simulink model "Provaa"  (R2020a)
settings: Solver=VariableStepAuto  StartTime=0.0  StopTime=10.0  RelTol=1e-3
libraries: simulink x1
settings Model: Creator=cvalo  LastModifiedBy=cvalo

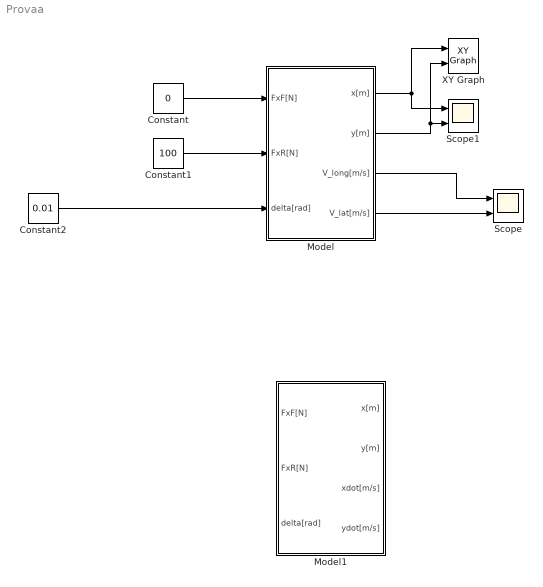
== system Provaa ==
  Constant : Constant  Value=0
  Constant1 : Constant  Value=100
  Constant2 : Constant  Value=0.01
  Model : Subsystem
  Model1 : Subsystem
  Scope : Scope  NumInputPorts=2
  Scope1 : Scope  NumInputPorts=2
  XY Graph : simulink/Sinks/XY Graph  xmin=-1  xmax=500  ymin=-10  ymax=250  st=-1
  wires:
  Model/3(V_long[m/s]) -> Scope/1
  Model/4(V_lat[m/s]) -> Scope/2
  Model/1(x[m]) -> Scope1/1, XY Graph/1
  Model/2(y[m]) -> XY Graph/2, Scope1/2
  Constant/1 -> Model/1(FxF[N])
  Constant1/1 -> Model/2(FxR[N])
  Constant2/1 -> Model/3(delta[rad])

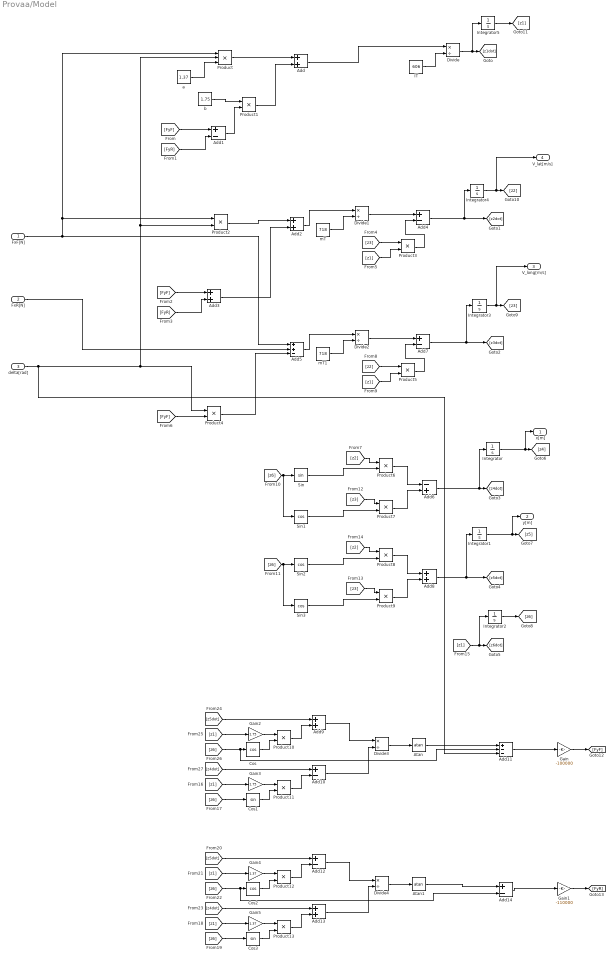
== system Provaa/Model ==
  FxF[N] : Inport  Unit=N
  FxR[N] : Inport  Port=2  Unit=N
  delta[rad] : Inport  Port=3  Unit=rad
  Add{,2..3,8..9,13} (6 alike) : Sum
  Add{1,4,7,10,12,14} (6 alike) : Sum  Inputs=+-
  Add11 : Sum  Inputs=+--
  Add5 : Sum  Inputs=++-
  Add6 : Sum  Inputs=-+
  Atan : Trigonometry  Operator=atan
  Atan1 : Trigonometry  Operator=atan
  Cos : Trigonometry  Operator=cos
  Cos1 : Trigonometry
  Cos2 : Trigonometry  Operator=cos
  Cos3 : Trigonometry
  Divide{,1..4} (5 alike) : Product  Inputs=*/
  Gain : Gain  Gain=-100000
  Gain1 : Gain  Gain=-110000
  Gain2 : Gain  Gain=1.75
  Gain3 : Gain  Gain=1.75
  Gain4 : Gain  Gain=1.37
  Gain5 : Gain  Gain=1.37
  IT : Constant  Value=606
  Integrator{,1..2,4..5} (5 alike) : Integrator
  Integrator3 : Integrator  InitialCondition=10
  Product : Product  Inputs=3
  Product{1..13} (13 alike) : Product
  Sin : Trigonometry
  Sin1 : Trigonometry  Operator=cos
  Sin2 : Trigonometry  Operator=cos
  Sin3 : Trigonometry  Operator=cos
  a : Constant  Value=1.37
  b : Constant  Value=1.75
  mT : Constant  Value=718
  mT1 : Constant  Value=718
  x[m] : Outport  Unit=m
  y[m] : Outport  Port=2  Unit=m
  V_long[m/s] : Outport  Port=3  Unit=m/s
  V_lat[m/s] : Outport  Port=4  Unit=m/s
  wires:
  Divide/1 -> Integrator5/1, [z1dot]
  IT/1 -> Divide/2
  a/1 -> Product/3
  Product/1 -> Add/1
  Product1/1 -> Add/2
  b/1 -> Product1/1
  Add1/1 -> Product1/2
  [FyF] -> Add1/1
  [FyR] -> Add1/2
  Add/1 -> Divide/1
  Add3/1 -> Add2/2
  [FyF] -> Add3/1
  Divide1/1 -> Add4/1
  Add2/1 -> Divide1/1
  [FyR] -> Add3/2
  mT/1 -> Divide1/2
  Product2/1 -> Add2/1
  Add4/1 -> Integrator4/1, [z2dot]
  Product3/1 -> Add4/2
  [z3] -> Product3/1
  [z1] -> Product3/2
  [z1] -> Product5/2
  FxF[N]/1 -> Add5/1, Product/1, Product2/1
  [FyF] -> Product4/2
  Product5/1 -> Add7/2
  Add5/1 -> Divide2/1
  Add7/1 -> Integrator3/1, [z3dot]
  Product4/1 -> Add5/3
  mT1/1 -> Divide2/2
  Divide2/1 -> Add7/1
  [z2] -> Product5/1
  FxR[N]/1 -> Add5/2
  Add6/1 -> Integrator/1, [z4dot]
  Product6/1 -> Add6/1
  Product7/1 -> Add6/2
  [z2] -> Product6/1
  Sin/1 -> Product6/2
  [z3] -> Product7/1
  Sin1/1 -> Product7/2
  [z6] -> Sin1/1, Sin/1
  Sin2/1 -> Product8/2
  Sin3/1 -> Product9/2
  Product8/1 -> Add8/1
  [z3] -> Product9/1
  Product9/1 -> Add8/2
  [z2] -> Product8/1
  [z6] -> Sin3/1, Sin2/1
  [z1] -> Integrator2/1, [z6dot]
  Integrator/1 -> x[m]/1, [z4]
  Integrator1/1 -> y[m]/1, [z5]
  Add8/1 -> [z5dot], Integrator1/1
  Integrator2/1 -> [z6]
  Integrator3/1 -> V_long[m/s]/1, [z3]
  Integrator4/1 -> V_lat[m/s]/1, [z2]
  Integrator5/1 -> [z1]
  Gain1/1 -> [FyR]
  Gain/1 -> [FyF]
  Atan/1 -> Add11/1
  Add9/1 -> Divide3/1
  Cos/1 -> Product10/2
  delta[rad]/1 -> Add11/3, Product4/1, Product/2, Product2/2
  [z4dot] -> Add10/1
  Add14/1 -> Gain1/1
  Cos3/1 -> Product13/2
  Divide3/1 -> Atan/1
  Product13/1 -> Add13/2
  Gain3/1 -> Product11/1
  Add10/1 -> Divide3/2
  [z5dot] -> Add9/1
  [z6] -> Cos1/1
  [z6] -> Add11/2, Cos/1
  [z6] -> Add14/2, Cos2/1
  Cos2/1 -> Product12/2
  [z1] -> Gain4/1
  Gain2/1 -> Product10/1
  Gain5/1 -> Product13/1
  Add11/1 -> Gain/1
  Divide4/1 -> Atan1/1
  Add12/1 -> Divide4/1
  [z1] -> Gain3/1
  Add13/1 -> Divide4/2
  Product10/1 -> Add9/2
  Cos1/1 -> Product11/2
  [z5dot] -> Add12/1
  Atan1/1 -> Add14/1
  [z1] -> Gain2/1
  [z6] -> Cos3/1
  Product11/1 -> Add10/2
  Product12/1 -> Add12/2
  [z1] -> Gain5/1
  Gain4/1 -> Product12/1
  [z4dot] -> Add13/1

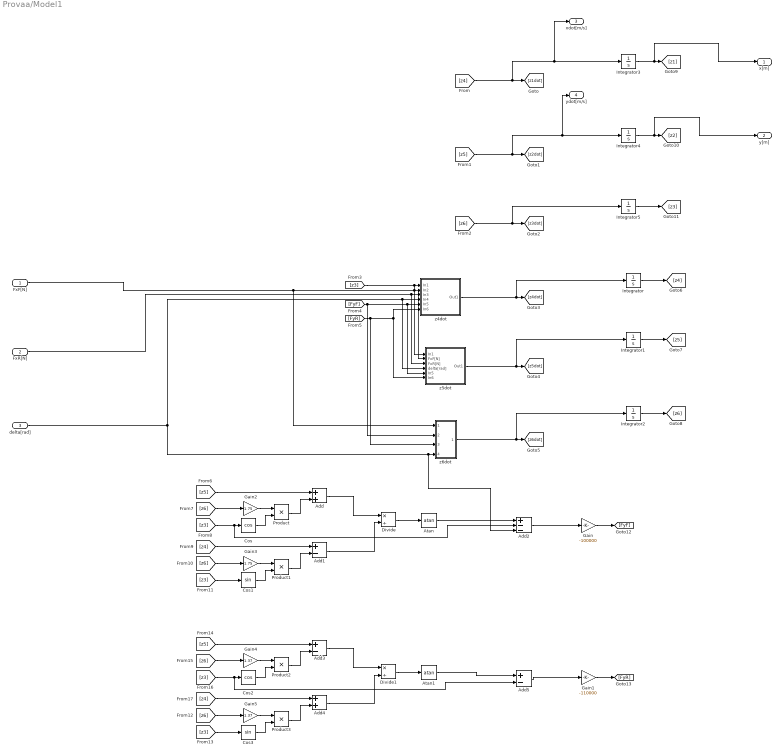
== system Provaa/Model1 ==
  FxF[N] : Inport  Unit=N
  FxR[N] : Inport  Port=2  Unit=N
  delta[rad] : Inport  Port=3  Unit=rad
  Add : Sum
  Add1 : Sum  Inputs=+-
  Add2 : Sum  Inputs=+--
  Add3 : Sum  Inputs=+-
  Add4 : Sum
  Add5 : Sum  Inputs=+-
  Atan : Trigonometry  Operator=atan
  Atan1 : Trigonometry  Operator=atan
  Cos : Trigonometry  Operator=cos
  Cos1 : Trigonometry
  Cos2 : Trigonometry  Operator=cos
  Cos3 : Trigonometry
  Divide : Product  Inputs=*/
  Divide1 : Product  Inputs=*/
  Gain : Gain  Gain=-100000
  Gain1 : Gain  Gain=-110000
  Gain2 : Gain  Gain=1.75
  Gain3 : Gain  Gain=1.75
  Gain4 : Gain  Gain=1.37
  Gain5 : Gain  Gain=1.37
  Integrator : Integrator  InitialCondition=10
  Integrator{1..5} (5 alike) : Integrator
  Product{,1..3} (4 alike) : Product
  z4dot : Subsystem
  z5dot : Subsystem
  z6dot : Subsystem
  x[m] : Outport  Unit=m
  y[m] : Outport  Port=2  Unit=m
  xdot[m/s] : Outport  Port=3  Unit=m/s
  ydot[m/s] : Outport  Port=4  Unit=m/s
  wires:
  [z3] -> z5dot/1(In1), z4dot/1(In1)
  FxF[N]/1 -> z6dot/1(In1), z5dot/2(FxF[N]), z4dot/2(In2)
  FxR[N]/1 -> z5dot/3(FxR[N]), z4dot/3(In3)
  delta[rad]/1 -> Add2/3, z6dot/4(In4), z4dot/4(In4), z5dot/4(delta[rad])
  [FyF] -> z6dot/2(In2), z4dot/5(In5), z5dot/5(In5)
  [FyR] -> z6dot/3(In3), z5dot/6(In6), z4dot/6(In6)
  z4dot/1(Out1) -> Integrator/1, [z4dot]
  Integrator/1 -> [z4]
  Integrator1/1 -> [z5]
  z5dot/1(Out1) -> Integrator1/1, [z5dot]
  Integrator2/1 -> [z6]
  z6dot/1(Out1) -> Integrator2/1, [z6dot]
  Integrator3/1 -> x[m]/1, [z1]
  [z4] -> xdot[m/s]/1, Integrator3/1, [z1dot]
  Integrator4/1 -> y[m]/1, [z2]
  [z5] -> ydot[m/s]/1, Integrator4/1, [z2dot]
  Integrator5/1 -> [z3]
  [z6] -> Integrator5/1, [z3dot]
  Gain/1 -> [FyF]
  Gain1/1 -> [FyR]
  Atan/1 -> Add2/1
  Divide/1 -> Atan/1
  [z5] -> Add/1
  Add/1 -> Divide/1
  [z6] -> Gain2/1
  Gain2/1 -> Product/1
  Cos/1 -> Product/2
  [z3] -> Add2/2, Cos/1
  Product/1 -> Add/2
  [z3] -> Cos1/1
  [z4] -> Add1/1
  Add1/1 -> Divide/2
  Product1/1 -> Add1/2
  Gain3/1 -> Product1/1
  [z6] -> Gain3/1
  Cos1/1 -> Product1/2
  Add2/1 -> Gain/1
  [z3] -> Add5/2, Cos2/1
  [z6] -> Gain5/1
  Add5/1 -> Gain1/1
  Product3/1 -> Add4/2
  Gain5/1 -> Product3/1
  Cos3/1 -> Product3/2
  [z4] -> Add4/1
  [z3] -> Cos3/1
  Atan1/1 -> Add5/1
  Add4/1 -> Divide1/2
  [z5] -> Add3/1
  Add3/1 -> Divide1/1
  Product2/1 -> Add3/2
  Gain4/1 -> Product2/1
  Divide1/1 -> Atan1/1
  [z6] -> Gain4/1
  Cos2/1 -> Product2/2

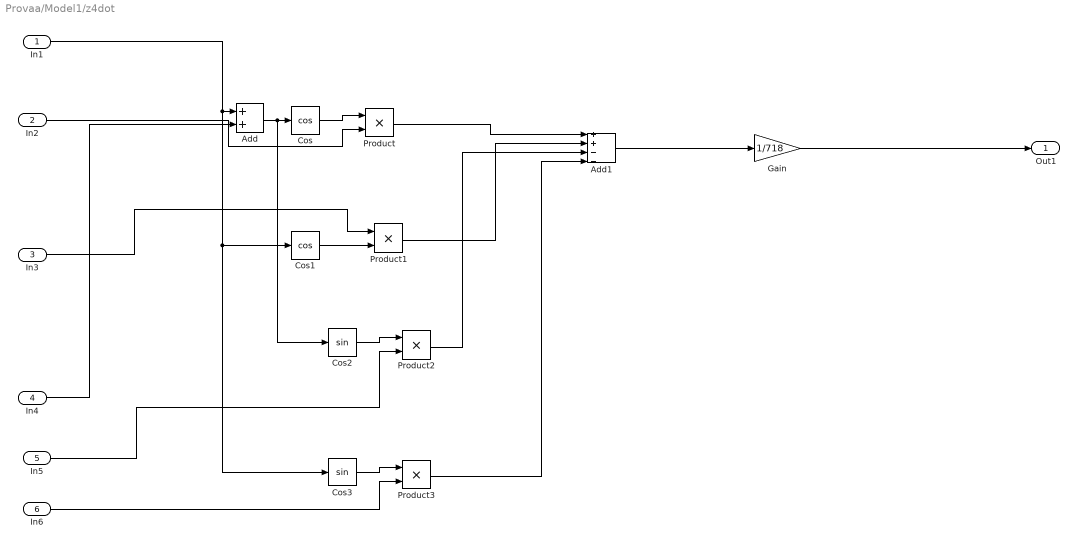
== system Provaa/Model1/z4dot ==
  In1 : Inport
  In2 : Inport  Port=2
  In3 : Inport  Port=3
  In4 : Inport  Port=4
  In5 : Inport  Port=5
  In6 : Inport  Port=6
  Add : Sum
  Add1 : Sum  Inputs=++--
  Cos : Trigonometry  Operator=cos
  Cos1 : Trigonometry  Operator=cos
  Cos2 : Trigonometry
  Cos3 : Trigonometry
  Gain : Gain  Gain=1/718
  Product{,1..3} (4 alike) : Product
  Out1 : Outport
  wires:
  In1/1 -> Cos1/1, Cos3/1, Add/1
  Gain/1 -> Out1/1
  Product2/1 -> Add1/3
  Cos1/1 -> Product1/2
  Add/1 -> Cos2/1, Cos/1
  Product3/1 -> Add1/4
  Cos2/1 -> Product2/1
  Cos/1 -> Product/1
  Add1/1 -> Gain/1
  Cos3/1 -> Product3/1
  Product1/1 -> Add1/2
  Product/1 -> Add1/1
  In6/1 -> Product3/2
  In4/1 -> Add/2
  In2/1 -> Product/2
  In3/1 -> Product1/1
  In5/1 -> Product2/2

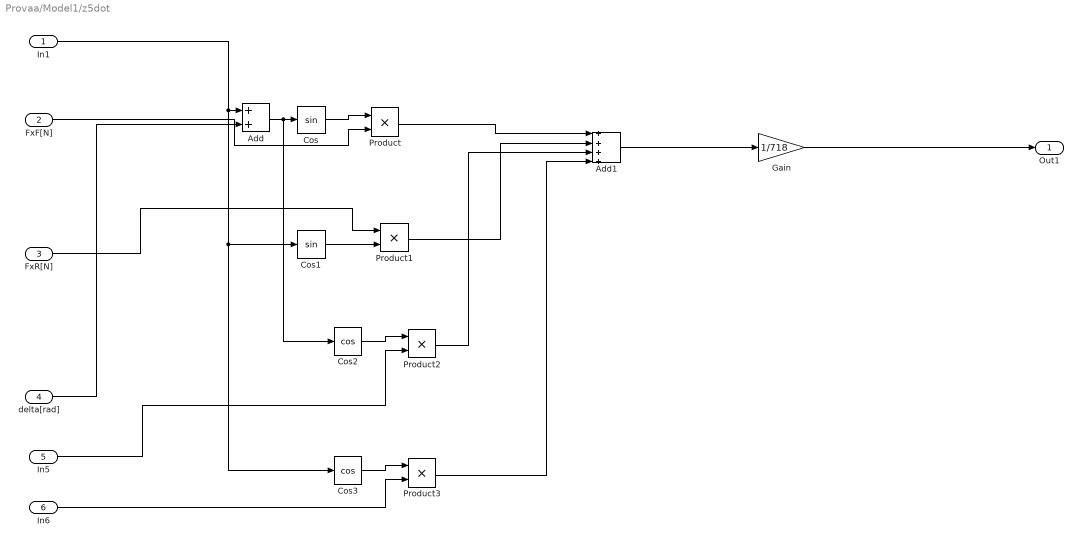
== system Provaa/Model1/z5dot ==
  In1 : Inport
  FxF[N] : Inport  Port=2
  FxR[N] : Inport  Port=3
  delta[rad] : Inport  Port=4
  In5 : Inport  Port=5
  In6 : Inport  Port=6
  Add : Sum
  Add1 : Sum  Inputs=++++
  Cos : Trigonometry
  Cos1 : Trigonometry
  Cos2 : Trigonometry  Operator=cos
  Cos3 : Trigonometry  Operator=cos
  Gain : Gain  Gain=1/718
  Product{,1..3} (4 alike) : Product
  Out1 : Outport
  wires:
  In1/1 -> Cos1/1, Cos3/1, Add/1
  Gain/1 -> Out1/1
  Product2/1 -> Add1/3
  Cos1/1 -> Product1/2
  Add/1 -> Cos2/1, Cos/1
  Product3/1 -> Add1/4
  Cos2/1 -> Product2/1
  Cos/1 -> Product/1
  Add1/1 -> Gain/1
  Cos3/1 -> Product3/1
  Product1/1 -> Add1/2
  Product/1 -> Add1/1
  In6/1 -> Product3/2
  delta[rad]/1 -> Add/2
  FxF[N]/1 -> Product/2
  FxR[N]/1 -> Product1/1
  In5/1 -> Product2/2

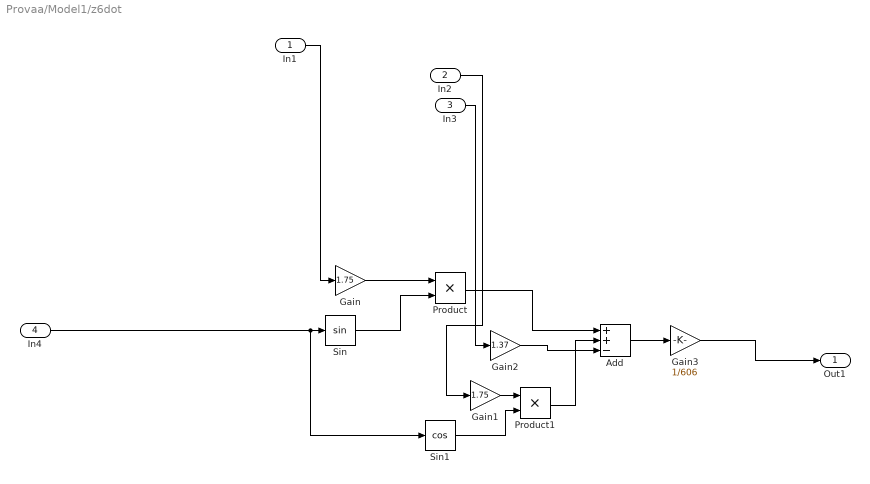
== system Provaa/Model1/z6dot ==
  In1 : Inport
  In2 : Inport  Port=2
  In3 : Inport  Port=3
  In4 : Inport  Port=4
  Add : Sum  Inputs=++-
  Gain : Gain  Gain=1.75
  Gain1 : Gain  Gain=1.75
  Gain2 : Gain  Gain=1.37
  Gain3 : Gain  Gain=1/606
  Product : Product
  Product1 : Product
  Sin : Trigonometry
  Sin1 : Trigonometry  Operator=cos
  Out1 : Outport
  wires:
  Sin1/1 -> Product1/2
  In4/1 -> Sin1/1, Sin/1
  Product/1 -> Add/1
  Gain1/1 -> Product1/1
  Add/1 -> Gain3/1
  Product1/1 -> Add/2
  Gain/1 -> Product/1
  Sin/1 -> Product/2
  Gain2/1 -> Add/3
  In3/1 -> Gain2/1
  Gain3/1 -> Out1/1
  In2/1 -> Gain1/1
  In1/1 -> Gain/1
